simulink model "sxem_711"  (R2023a)
settings: Solver=VariableStepAuto  StartTime=0.0  StopTime=50.0  RelTol=1e-3
settings Model: Creator=User  LastModifiedBy=User

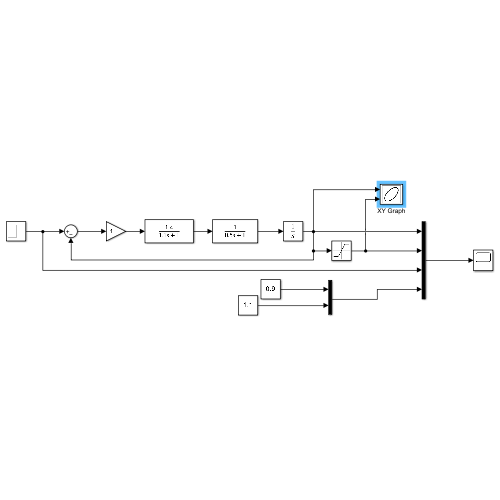
[thumbnail: Simulink's stored preview of the top-level diagram]
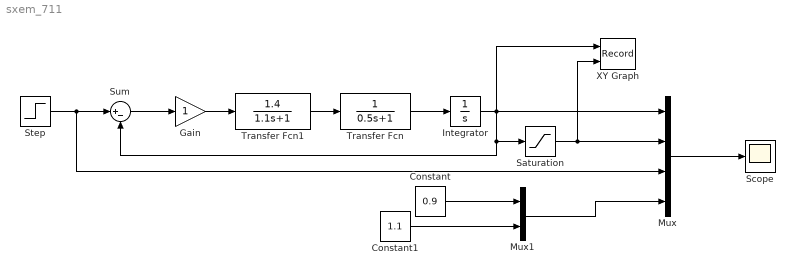
== system sxem_711 ==
  Constant : Constant  Value=0.9
  Constant1 : Constant  Value=1.1
  Gain : Gain
  Integrator : Integrator
  Mux : Mux
  Mux1 : Mux  Inputs=2
  Saturation : Saturate  UpperLimit=1.1  LowerLimit=0.9
  Scope : Scope
  Step : Step  Time=0  SampleTime=0
  Sum : Sum  Inputs=|+-
  Transfer Fcn : TransferFcn  Denominator=[0.5 1]
  Transfer Fcn1 : TransferFcn  Numerator=[1.4]  Denominator=[1.1 1]
  XY Graph : Record  FileSettingsInternal="{\"entries\":[{\"content\":{\"excelSettings\":{\"content\":{},\"type\":\"Streamout.ExcelSettings\"}},\"type\":\"Streamout.FileSettingStorage\",\"uuid\":\"\"}],\"packageUris\":[\"http:\\/\\/schema.mathworks.com\\/mf0\\/streamout_blocks\\/R2020a\"],\"version\":\"1.0\"}"  Layout=[1 1]  SignalsInternal="{\"entries\":[{\"content\":{\"signals\":[{\"content\":{\"blockPath\":[],\"dimensions\":[1],\"domain\":\"\",\"lineColor\":\"#a2142f\",\"plots\":[1],\"port\":1,\"sid\":[\"\"],\"signalID\":100,\"signalName\":\"Integrator\"},\"type\":\"RecordBlkView.Signal\",\"uuid\":\"\"},{\"content\":{\"blockPath\":[],\"dimensions\":[1],\"domain\":\"\",\"lineColor\":\"#139fff\",\"plots\":[1],\"port\":2,\"sid\":[\"\"],\"signalID\":104,\"signalName\":\"Saturation\"},\"type\":\"RecordBlkView.Signal\",\"uuid\":\"\"}]},\"type\":\"RecordBlkView.InputSignals\",\"uuid\":\"\"}],\"packageUris\":[\"http:\\/\\/schema.mathworks.com\\/mf0\\/streamout_blocks\\/R2020a\"],\"version\":\"1.0\"}"  VisualizationBindings="{\"xyplotplugin\":{\"info\":[{\"series\":[{\"bindingParametersList\":[{\"parameter\":\"Y-Axis\",\"signalID\":104,\"signalName\":\"Saturation\"},{\"parameter\":\"X-Axis\",\"signalID\":100,\"signalName\":\"Integrator\"}],\"seriesID\":27353}],\"subplotID\":1}]}}"  CompatibilityTag=XY
  wires:
  Mux/1 -> Scope/1
  Transfer Fcn1/1 -> Transfer Fcn/1
  Gain/1 -> Transfer Fcn1/1
  Sum/1 -> Gain/1
  Step/1 -> Mux/3, Sum/1
  Integrator/1 -> XY Graph/1, Sum/2, Saturation/1, Mux/1
  Transfer Fcn/1 -> Integrator/1
  Saturation/1 -> XY Graph/2, Mux/2
  Constant1/1 -> Mux1/2
  Constant/1 -> Mux1/1
  Mux1/1 -> Mux/4
